simulink library "lib_startup_procedure"  (R2023a)
settings: Solver=VariableStepAuto  StartTime=0.0  StopTime=10.0  RelTol=1e-3
undefined symbols (not defined in the file): bit, lb_parSampTime
libraries: simulink x4, lib_conversion x2, lib_discrete_time_integrator x2
settings Model: Creator=cav2ofo  LastModifiedBy=lenovo
settings OptimizationCC: ReuseModelBlockBuffer=off

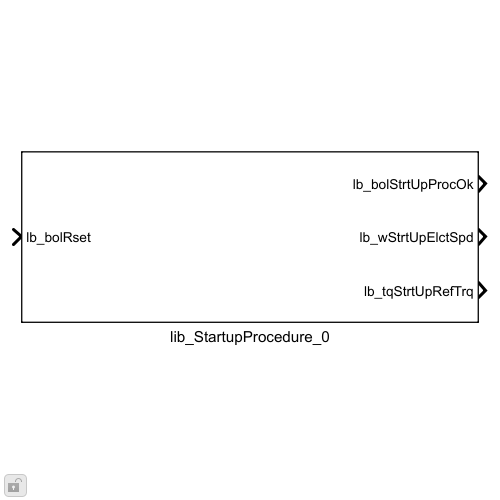
[thumbnail: Simulink's stored preview of the top-level diagram]
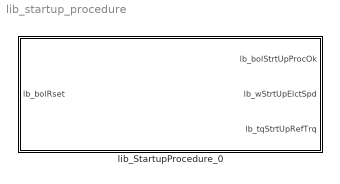
== system lib_startup_procedure ==
  lib_StartupProcedure_0 : Subsystem  mask{lb_parSampTime=2e-3, lb_parStrtUpSpdRampCoef=2000, lb_parStrtUpTrqRampCoef=30, lb_parStrtUpSpd=200, lb_parStrtUpTrq=0.6, lb_parSpdRampCoefMaxVal=10000*5*pi/30, lb_parSpdRampCoefMinVal=-10000*5*pi/30, lb_parTrqRampCoefMaxVal=30, lb_parTrqRampCoefMinVal=-30, lb_parMaxSampTime=lb_parSampTime, lb_parMaxIntgGain=0, lb_parIntgScopMode=Generic signal, lb_parSatFlag=on, lb_parSpdAccmDataTypeMode=32-bit, lb_parTrqAccmDataTypeMode=32-bit, lb_parElctSpdDataType=fixdt(1,16,2^0,0), lb_parTrqDataType=fixdt(1,16,2^0,0)}
      mask prompts: lb_parSampTime "Sampling time [s]:"; lb_parStrtUpSpdRampCoef "Ramp coefficient of startup electric speed [rad/s2]:"; lb_parStrtUpTrqRampCoef "Ramp coefficient of startup torque [Nm/s]:"; lb_parStrtUpSpd "Start up electric speed [rad/s]:"; lb_parStrtUpTrq "Start up torque [Nm]:"; lb_parSpdRampCoefMaxVal "Maximum ramp coefficient of startup speed [rad/s2]:"; lb_parSpdRampCoefMinVal "Minimum ramp coefficient of startup speed [rad/s2]:"; lb_parTrqRampCoefMaxVal "Maximum ramp coefficient of startup torque [Nm/s]:"; lb_parTrqRampCoefMinVal "Minimum ramp coefficient of startup torque [Nm/s]:"; lb_parMaxSampTime "Maximum sampling time [s]:"; lb_parMaxIntgGain "Maximum integral gain [ou/(iu*s)]:"; lb_parIntgScopMode "Integration scope:"; lb_parSatFlag "Output saturation"; lb_parSpdAccmDataTypeMode "Accumulator data type mode for speed:"; lb_parTrqAccmDataTypeMode "Accumulator data type mode for torque:"; lb_parElctSpdDataType "Electric speed data type:"; lb_parTrqDataType "Torque data type:"
      mask init:
      | lb_parMaxSampTime = double(lb_parSampTime);
      mask TypeOptions lb_parSpdRampCoefMaxVal: lib_DiscreteTimeIntegrator_1/lb_parMaxInpVal
      mask TypeOptions lb_parSpdRampCoefMinVal: lib_DiscreteTimeIntegrator_1/lb_parMinInpVal
      mask TypeOptions lb_parTrqRampCoefMaxVal: lib_DiscreteTimeIntegrator_2/lb_parMaxInpVal
      mask TypeOptions lb_parTrqRampCoefMinVal: lib_DiscreteTimeIntegrator_2/lb_parMinInpVal
      mask TypeOptions lb_parMaxSampTime: lib_DiscreteTimeIntegrator_1/lb_parMaxSampTime | lib_DiscreteTimeIntegrator_2/lb_parMaxSampTime
      mask TypeOptions lb_parMaxIntgGain: lib_DiscreteTimeIntegrator_1/lb_parMaxIntgGain | lib_DiscreteTimeIntegrator_2/lb_parMaxIntgGain
      mask TypeOptions lb_parIntgScopMode: lib_DiscreteTimeIntegrator_1/lb_parIntgScopMode | lib_DiscreteTimeIntegrator_2/lb_parIntgScopMode
      mask TypeOptions lb_parSatFlag: lib_DiscreteTimeIntegrator_1/lb_parSatFlag | lib_DiscreteTimeIntegrator_2/lb_parSatFlag
      mask TypeOptions lb_parSpdAccmDataTypeMode: lib_DiscreteTimeIntegrator_1/lb_parAccmDataTypeMode
      mask TypeOptions lb_parTrqAccmDataTypeMode: lib_DiscreteTimeIntegrator_2/lb_parAccmDataTypeMode
      mask TypeOptions lb_parElctSpdDataType: lib_DiscreteTimeIntegrator_1/lb_parOutpDataType
      mask TypeOptions lb_parTrqDataType: lib_DiscreteTimeIntegrator_2/lb_parOutpDataType
      mask DialogControl DescGroupVar Prompt: VHIT control library
      mask DialogControl DescTextVar Prompt: Start up procedure
      mask DialogControl Container3 Prompt: Data types:

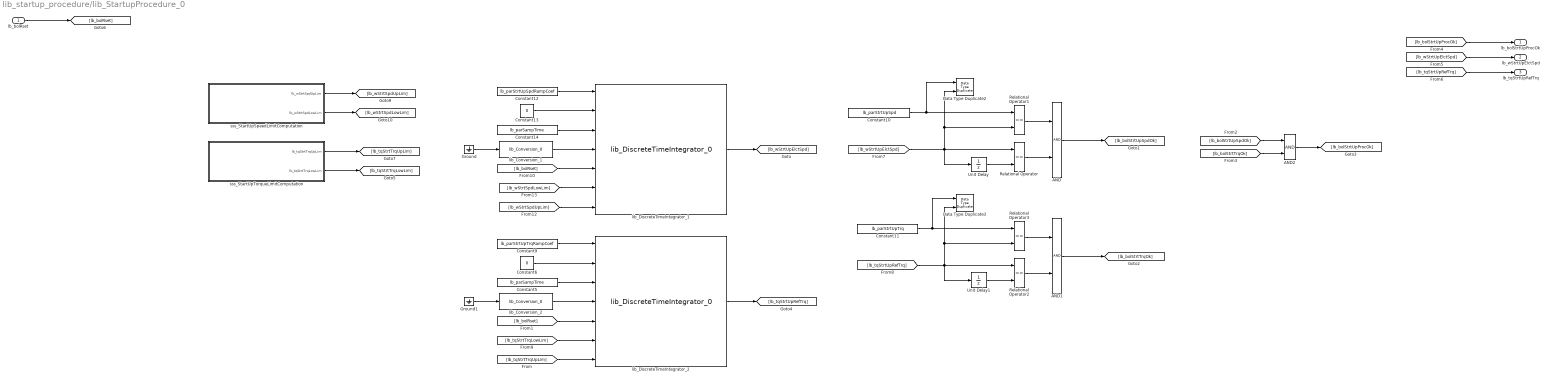
== system lib_startup_procedure/lib_StartupProcedure_0 ==
  lb_bolRset : Inport
  AND : Logic  AllPortsSameDT=off  OutDataTypeStr=boolean
  AND1 : Logic  AllPortsSameDT=off  OutDataTypeStr=boolean
  AND2 : Logic  AllPortsSameDT=off  OutDataTypeStr=boolean
  Constant10 : Constant  Value=lb_parStrtUpSpd  OutDataTypeStr=Inherit: Inherit via back propagation
  Constant11 : Constant  Value=lb_parStrtUpTrq  OutDataTypeStr=Inherit: Inherit via back propagation
  Constant12 : Constant  Value=lb_parStrtUpSpdRampCoef
  Constant13 : Constant  Value=0  OutDataTypeStr=lb_parElctSpdDataType
  Constant14 : Constant  Value=lb_parSampTime
  Constant5 : Constant  Value=lb_parSampTime
  Constant6 : Constant  Value=0  OutDataTypeStr=lb_parTrqDataType
  Constant9 : Constant  Value=lb_parStrtUpTrqRampCoef
  Data Type Duplicate2 : DataTypeDuplicate
  Data Type Duplicate3 : DataTypeDuplicate
  Ground : Ground
  Ground1 : Ground
  Relational Operator{,1..3} (4 alike) : RelationalOperator  Operator===  OutDataTypeStr=boolean  RndMeth=Simplest  InputSameDT=off
  Unit Delay : UnitDelay  SampleTime=-1  HasFrameUpgradeWarning=on
  Unit Delay1 : UnitDelay  SampleTime=-1  HasFrameUpgradeWarning=on
  lib_Conversion_1 : lib_conversion/lib_Conversion_0  lb_parDataType=uint8  lb_parOutpMaxVal=[]  lb_parOutpMinVal=[]  lb_parSatFlag=off
  lib_Conversion_2 : lib_conversion/lib_Conversion_0  lb_parDataType=uint8  lb_parOutpMaxVal=[]  lb_parOutpMinVal=[]  lb_parSatFlag=off
  lib_DiscreteTimeIntegrator_1 : lib_discrete_time_integrator/lib_DiscreteTimeIntegrator_0  lb_parMaxInpVal=lb_parSpdRampCoefMaxVal  lb_parMinInpVal=lb_parSpdRampCoefMinVal  lb_parMaxSampTime=lb_parMaxSampTime  lb_parMaxIntgGain=lb_parMaxIntgGain  lb_parAccmDataTypeMode=32-bit  lb_parOutpDataType=fixdt(1,16,2^0,0)  lb_parIntgScopMode=Generic signal  lb_parSatFlag=on
  lib_DiscreteTimeIntegrator_2 : lib_discrete_time_integrator/lib_DiscreteTimeIntegrator_0  lb_parMaxInpVal=lb_parTrqRampCoefMaxVal  lb_parMinInpVal=lb_parTrqRampCoefMinVal  lb_parMaxSampTime=lb_parMaxSampTime  lb_parMaxIntgGain=lb_parMaxIntgGain  lb_parAccmDataTypeMode=32-bit  lb_parOutpDataType=fixdt(1,16,2^0,0)  lb_parIntgScopMode=Generic signal  lb_parSatFlag=on
  sss_StartUpSpeedLimitComputation : Subsystem
  sss_StartUpTorqueLimitComputation : Subsystem
  lb_bolStrtUpProcOk : Outport
  lb_wStrtUpElctSpd : Outport  Port=2
  lb_tqStrtUpRefTrq : Outport  Port=3
  wires:
  Constant6/1 -> lib_DiscreteTimeIntegrator_2/2
  Constant9/1 -> lib_DiscreteTimeIntegrator_2/1
  lb_bolRset/1 -> [lb_bolRset]
  [lb_wStrtUpElctSpd] -> Data Type Duplicate2/2, Relational Operator1/2, Relational Operator/1, Unit Delay/1
  Unit Delay/1 -> Relational Operator/2
  Relational Operator/1 -> AND/2
  Constant10/1 -> Data Type Duplicate2/1, Relational Operator1/1
  Relational Operator1/1 -> AND/1
  Relational Operator2/1 -> AND1/2
  Relational Operator3/1 -> AND1/1
  Unit Delay1/1 -> Relational Operator2/2
  [lb_tqStrtUpRefTrq] -> Data Type Duplicate3/2, Relational Operator3/2, Relational Operator2/1, Unit Delay1/1
  Constant11/1 -> Data Type Duplicate3/1, Relational Operator3/1
  AND/1 -> [lb_bolStrtUpSpdOk]
  AND1/1 -> [lb_bolStrtTrqOk]
  [lb_bolStrtTrqOk] -> AND2/2
  [lb_bolStrtUpSpdOk] -> AND2/1
  AND2/1 -> [lb_bolStrtUpProcOk]
  [lb_bolStrtUpProcOk] -> lb_bolStrtUpProcOk/1
  [lb_tqStrtUpRefTrq] -> lb_tqStrtUpRefTrq/1
  [lb_wStrtUpElctSpd] -> lb_wStrtUpElctSpd/1
  lib_DiscreteTimeIntegrator_1/1 -> [lb_wStrtUpElctSpd]
  lib_DiscreteTimeIntegrator_2/1 -> [lb_tqStrtUpRefTrq]
  Constant12/1 -> lib_DiscreteTimeIntegrator_1/1
  Constant13/1 -> lib_DiscreteTimeIntegrator_1/2
  Constant14/1 -> lib_DiscreteTimeIntegrator_1/3
  [lb_bolRset] -> lib_DiscreteTimeIntegrator_1/5
  lib_Conversion_1/1 -> lib_DiscreteTimeIntegrator_1/4
  Ground/1 -> lib_Conversion_1/1
  sss_StartUpSpeedLimitComputation/2(lb_wStrtSpdLowLim) -> [lb_wStrtSpdLowLim]
  sss_StartUpSpeedLimitComputation/1(lb_wStrtSpdUpLim) -> [lb_wStrtSpdUpLim]
  [lb_wStrtSpdUpLim] -> lib_DiscreteTimeIntegrator_1/7
  [lb_wStrtSpdLowLim] -> lib_DiscreteTimeIntegrator_1/6
  Constant5/1 -> lib_DiscreteTimeIntegrator_2/3
  [lb_bolRset] -> lib_DiscreteTimeIntegrator_2/5
  sss_StartUpTorqueLimitComputation/1(lb_tqStrtTrqUpLim) -> [lb_tqStrtTrqUpLim]
  sss_StartUpTorqueLimitComputation/2(lb_tqStrtTrqLowLim) -> [lb_tqStrtTrqLowLim]
  [lb_tqStrtTrqUpLim] -> lib_DiscreteTimeIntegrator_2/7
  [lb_tqStrtTrqLowLim] -> lib_DiscreteTimeIntegrator_2/6
  Ground1/1 -> lib_Conversion_2/1
  lib_Conversion_2/1 -> lib_DiscreteTimeIntegrator_2/4

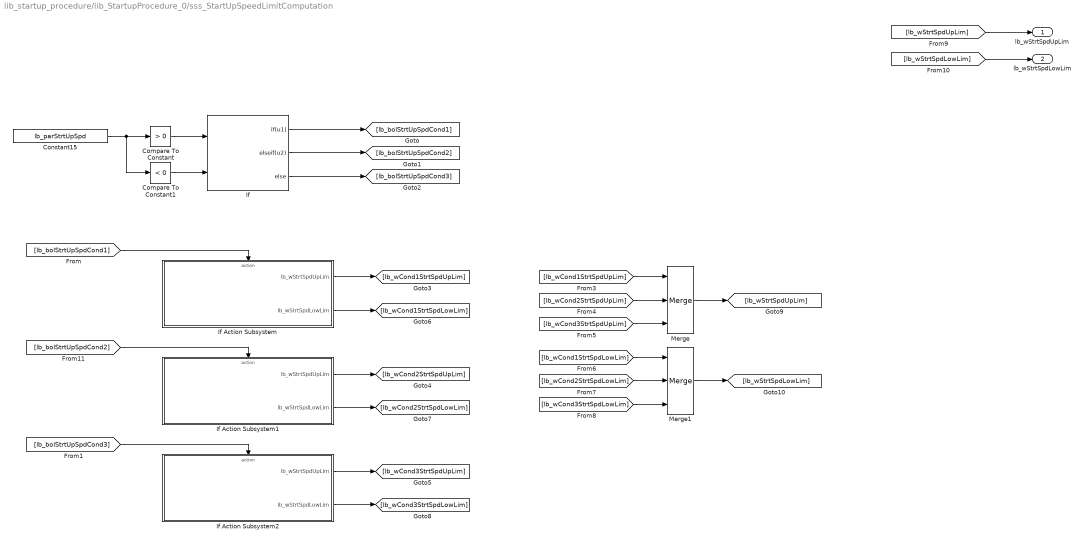
== system lib_startup_procedure/lib_StartupProcedure_0/sss_StartUpSpeedLimitComputation ==
  Compare To Constant : simulink/Logic and Bit Operations/Compare To Constant  relop=>  const=0  OutDataTypeStr=boolean
  Compare To Constant1 : simulink/Logic and Bit Operations/Compare To Constant  relop=<  const=0  OutDataTypeStr=boolean
  Constant15 : Constant  Value=lb_parStrtUpSpd
  If : If  NumInputs=2  IfExpression=u1  ElseIfExpressions=u2
  If Action Subsystem : Subsystem  TreatAsAtomicUnit=on
  If Action Subsystem1 : Subsystem  TreatAsAtomicUnit=on
  If Action Subsystem2 : Subsystem  TreatAsAtomicUnit=on
  Merge : Merge  Inputs=3
  Merge1 : Merge  Inputs=3
  lb_wStrtSpdUpLim : Outport
  lb_wStrtSpdLowLim : Outport  Port=2
  wires:
  Constant15/1 -> Compare To Constant1/1, Compare To Constant/1
  Compare To Constant/1 -> If/1
  Compare To Constant1/1 -> If/2
  If/1 -> [lb_bolStrtUpSpdCond1]
  [lb_bolStrtUpSpdCond1] -> If Action Subsystem/Action
  If/2 -> [lb_bolStrtUpSpdCond2]
  [lb_bolStrtUpSpdCond2] -> If Action Subsystem1/Action
  If/3 -> [lb_bolStrtUpSpdCond3]
  [lb_bolStrtUpSpdCond3] -> If Action Subsystem2/Action
  If Action Subsystem/1(lb_wStrtSpdUpLim) -> [lb_wCond1StrtSpdUpLim]
  If Action Subsystem1/1(lb_wStrtSpdUpLim) -> [lb_wCond2StrtSpdUpLim]
  If Action Subsystem2/1(lb_wStrtSpdUpLim) -> [lb_wCond3StrtSpdUpLim]
  If Action Subsystem/2(lb_wStrtSpdLowLim) -> [lb_wCond1StrtSpdLowLim]
  If Action Subsystem1/2(lb_wStrtSpdLowLim) -> [lb_wCond2StrtSpdLowLim]
  If Action Subsystem2/2(lb_wStrtSpdLowLim) -> [lb_wCond3StrtSpdLowLim]
  [lb_wCond1StrtSpdUpLim] -> Merge/1
  [lb_wCond2StrtSpdUpLim] -> Merge/2
  [lb_wCond3StrtSpdUpLim] -> Merge/3
  [lb_wCond1StrtSpdLowLim] -> Merge1/1
  [lb_wCond2StrtSpdLowLim] -> Merge1/2
  [lb_wCond3StrtSpdLowLim] -> Merge1/3
  [lb_wStrtSpdUpLim] -> lb_wStrtSpdUpLim/1
  [lb_wStrtSpdLowLim] -> lb_wStrtSpdLowLim/1
  Merge/1 -> [lb_wStrtSpdUpLim]
  Merge1/1 -> [lb_wStrtSpdLowLim]

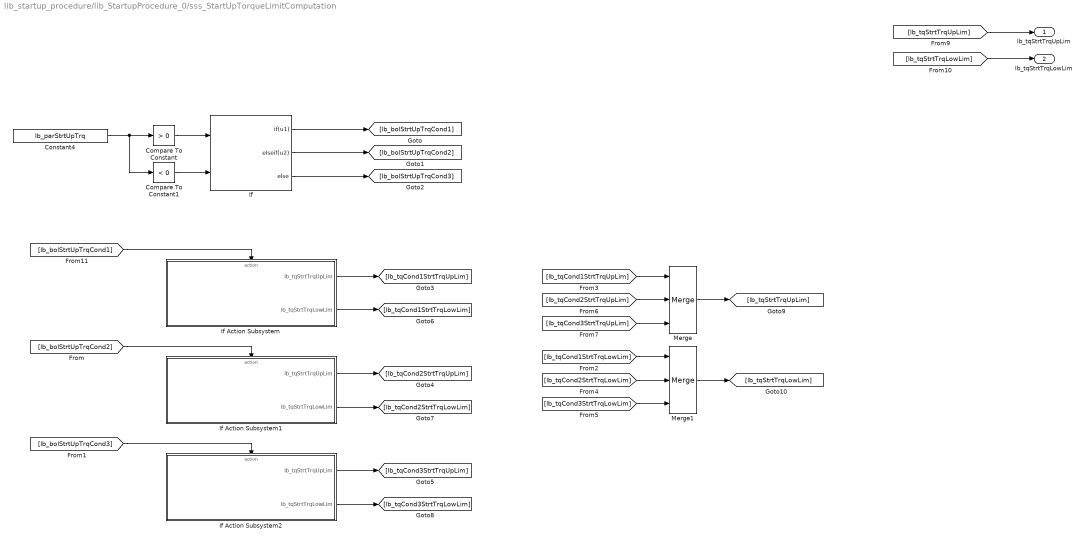
== system lib_startup_procedure/lib_StartupProcedure_0/sss_StartUpTorqueLimitComputation ==
  Compare To Constant : simulink/Logic and Bit Operations/Compare To Constant  relop=>  const=0  OutDataTypeStr=boolean
  Compare To Constant1 : simulink/Logic and Bit Operations/Compare To Constant  relop=<  const=0  OutDataTypeStr=boolean
  Constant4 : Constant  Value=lb_parStrtUpTrq
  If : If  NumInputs=2  IfExpression=u1  ElseIfExpressions=u2
  If Action Subsystem : Subsystem  TreatAsAtomicUnit=on
  If Action Subsystem1 : Subsystem  TreatAsAtomicUnit=on
  If Action Subsystem2 : Subsystem  TreatAsAtomicUnit=on
  Merge : Merge  Inputs=3
  Merge1 : Merge  Inputs=3
  lb_tqStrtTrqUpLim : Outport
  lb_tqStrtTrqLowLim : Outport  Port=2
  wires:
  Constant4/1 -> Compare To Constant1/1, Compare To Constant/1
  Compare To Constant/1 -> If/1
  Compare To Constant1/1 -> If/2
  If/1 -> [lb_bolStrtUpTrqCond1]
  [lb_bolStrtUpTrqCond1] -> If Action Subsystem/Action
  If/2 -> [lb_bolStrtUpTrqCond2]
  [lb_bolStrtUpTrqCond2] -> If Action Subsystem1/Action
  If/3 -> [lb_bolStrtUpTrqCond3]
  [lb_bolStrtUpTrqCond3] -> If Action Subsystem2/Action
  If Action Subsystem/1(lb_tqStrtTrqUpLim) -> [lb_tqCond1StrtTrqUpLim]
  If Action Subsystem1/1(lb_tqStrtTrqUpLim) -> [lb_tqCond2StrtTrqUpLim]
  If Action Subsystem2/1(lb_tqStrtTrqUpLim) -> [lb_tqCond3StrtTrqUpLim]
  If Action Subsystem/2(lb_tqStrtTrqLowLim) -> [lb_tqCond1StrtTrqLowLim]
  If Action Subsystem1/2(lb_tqStrtTrqLowLim) -> [lb_tqCond2StrtTrqLowLim]
  If Action Subsystem2/2(lb_tqStrtTrqLowLim) -> [lb_tqCond3StrtTrqLowLim]
  [lb_tqCond1StrtTrqUpLim] -> Merge/1
  [lb_tqCond2StrtTrqUpLim] -> Merge/2
  [lb_tqCond3StrtTrqUpLim] -> Merge/3
  [lb_tqCond1StrtTrqLowLim] -> Merge1/1
  [lb_tqCond2StrtTrqLowLim] -> Merge1/2
  [lb_tqCond3StrtTrqLowLim] -> Merge1/3
  [lb_tqStrtTrqUpLim] -> lb_tqStrtTrqUpLim/1
  [lb_tqStrtTrqLowLim] -> lb_tqStrtTrqLowLim/1
  Merge/1 -> [lb_tqStrtTrqUpLim]
  Merge1/1 -> [lb_tqStrtTrqLowLim]

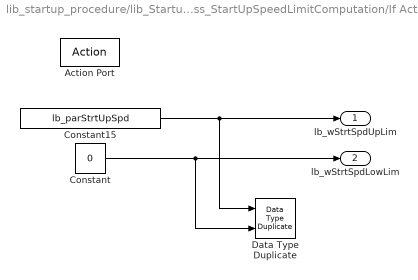
== system lib_startup_procedure/lib_StartupProcedure_0/sss_StartUpSpeedLimitComputation/If Action Subsystem ==
  Action Port : ActionPort
  Constant : Constant  Value=0  OutDataTypeStr=Inherit: Inherit via back propagation
  Constant15 : Constant  Value=lb_parStrtUpSpd
  Data Type Duplicate : DataTypeDuplicate
  lb_wStrtSpdUpLim : Outport
  lb_wStrtSpdLowLim : Outport  Port=2
  wires:
  Constant15/1 -> Data Type Duplicate/1, lb_wStrtSpdUpLim/1
  Constant/1 -> Data Type Duplicate/2, lb_wStrtSpdLowLim/1

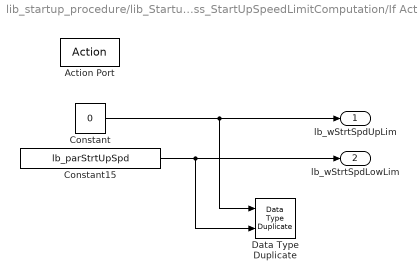
== system lib_startup_procedure/lib_StartupProcedure_0/sss_StartUpSpeedLimitComputation/If Action Subsystem1 ==
  Action Port : ActionPort
  Constant : Constant  Value=0  OutDataTypeStr=Inherit: Inherit via back propagation
  Constant15 : Constant  Value=lb_parStrtUpSpd
  Data Type Duplicate : DataTypeDuplicate
  lb_wStrtSpdUpLim : Outport
  lb_wStrtSpdLowLim : Outport  Port=2
  wires:
  Constant/1 -> Data Type Duplicate/1, lb_wStrtSpdUpLim/1
  Constant15/1 -> Data Type Duplicate/2, lb_wStrtSpdLowLim/1

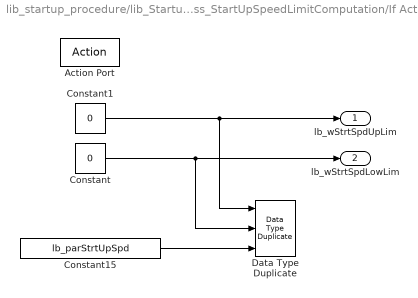
== system lib_startup_procedure/lib_StartupProcedure_0/sss_StartUpSpeedLimitComputation/If Action Subsystem2 ==
  Action Port : ActionPort
  Constant : Constant  Value=0  OutDataTypeStr=Inherit: Inherit via back propagation
  Constant1 : Constant  Value=0  OutDataTypeStr=Inherit: Inherit via back propagation
  Constant15 : Constant  Value=lb_parStrtUpSpd
  Data Type Duplicate : DataTypeDuplicate  NumInputPorts=3
  lb_wStrtSpdUpLim : Outport
  lb_wStrtSpdLowLim : Outport  Port=2
  wires:
  Constant1/1 -> Data Type Duplicate/1, lb_wStrtSpdUpLim/1
  Constant/1 -> Data Type Duplicate/2, lb_wStrtSpdLowLim/1
  Constant15/1 -> Data Type Duplicate/3

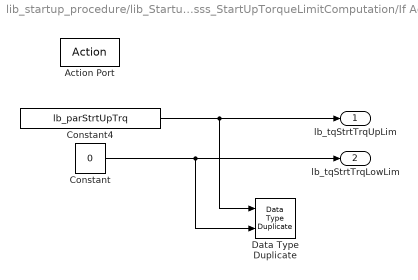
== system lib_startup_procedure/lib_StartupProcedure_0/sss_StartUpTorqueLimitComputation/If Action Subsystem ==
  Action Port : ActionPort
  Constant : Constant  Value=0  OutDataTypeStr=Inherit: Inherit via back propagation
  Constant4 : Constant  Value=lb_parStrtUpTrq
  Data Type Duplicate : DataTypeDuplicate
  lb_tqStrtTrqUpLim : Outport
  lb_tqStrtTrqLowLim : Outport  Port=2
  wires:
  Constant4/1 -> Data Type Duplicate/1, lb_tqStrtTrqUpLim/1
  Constant/1 -> Data Type Duplicate/2, lb_tqStrtTrqLowLim/1

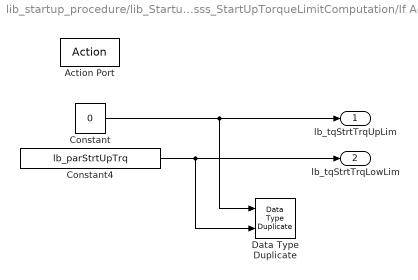
== system lib_startup_procedure/lib_StartupProcedure_0/sss_StartUpTorqueLimitComputation/If Action Subsystem1 ==
  Action Port : ActionPort
  Constant : Constant  Value=0  OutDataTypeStr=Inherit: Inherit via back propagation
  Constant4 : Constant  Value=lb_parStrtUpTrq
  Data Type Duplicate : DataTypeDuplicate
  lb_tqStrtTrqUpLim : Outport
  lb_tqStrtTrqLowLim : Outport  Port=2
  wires:
  Constant/1 -> Data Type Duplicate/1, lb_tqStrtTrqUpLim/1
  Constant4/1 -> Data Type Duplicate/2, lb_tqStrtTrqLowLim/1

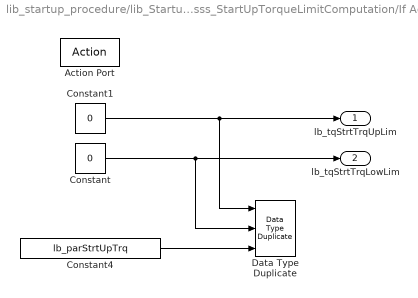
== system lib_startup_procedure/lib_StartupProcedure_0/sss_StartUpTorqueLimitComputation/If Action Subsystem2 ==
  Action Port : ActionPort
  Constant : Constant  Value=0  OutDataTypeStr=Inherit: Inherit via back propagation
  Constant1 : Constant  Value=0  OutDataTypeStr=Inherit: Inherit via back propagation
  Constant4 : Constant  Value=lb_parStrtUpTrq
  Data Type Duplicate : DataTypeDuplicate  NumInputPorts=3
  lb_tqStrtTrqUpLim : Outport
  lb_tqStrtTrqLowLim : Outport  Port=2
  wires:
  Constant1/1 -> Data Type Duplicate/1, lb_tqStrtTrqUpLim/1
  Constant/1 -> Data Type Duplicate/2, lb_tqStrtTrqLowLim/1
  Constant4/1 -> Data Type Duplicate/3
